simulink model "s8_10"  (Simulink 10.0)
settings: Solver=ode23  StartTime=0.0  StopTime=t_d  MaxStep=Tc  RelTol=1e-8  AbsTol=1e-8
values from neighbouring files (symbols this model uses):
  a = [1;1]    [MOTIONCONTROL.m]    (also in Robot_Maker.m = evalin('base', 'a'))
  F_v = K_r*diag([0.01 0.01])*K_r    [MOTIONCONTROL.m]
  g = [atan2d(r32,-r31);atan2d(sqrt(power(r13,2)+power(r23,2)),r33);atan2d(r23,r13)]    [DEMOGUI.m]    (also in MOTIONCONTROL.m = 9.81; invJacob_3axis.m = true; inverse_kinematics_Jac.m = true)
  K_d = 750*diag([1 1])    [MOTIONCONTROL.m]
  K_p = 375*diag([1 1])    [MOTIONCONTROL.m]
  pi_l = pi_m    [MOTIONCONTROL.m]
  q_d = [q1des q2des]    [MOTIONCONTROL.m]
  q_i = [q1ini q2ini]    [MOTIONCONTROL.m]
  Tc = 0.01    [MOTIONCONTROL.m]
  Ts = Tc    (= 0.01)    [MOTIONCONTROL.m]
undefined symbols (not defined in the file or in its folder): iner_l, pi_m
settings Model: Creator=luigivillani  LastModifiedBy=vivek  ExtModeAutoUpdateStatusClock=off
settings SolverCC: AutoScaleAbsTol=off  InitialStep=0.1*Tc
settings DataIOCC: SignalLoggingSaveFormat=ModelDataLogs  SaveOutput=off  SaveTime=off
settings OptimizationCC: BlockReduction=off  BooleanDataType=off  ExpressionDepthLimit=2147483647  InitFltsAndDblsToZero=on
settings DebuggingCC: SaveWithParameterizedLinksMsg=none  SignalResolutionControl=TryResolveAllWithWarning  MultiTaskDSMMsg=warning  MultiTaskCondExecSysMsg=none  FcnCallInpInsideContextMsg=warning  StateNameClashWarn=warning
settings HardwareCC: TargetUnknown=on
settings SFSimCC: SimUseLocalCustomCode=on  CustomCodeUndefinedFunction=FilterOut
settings RTWCC: RTWUseLocalCustomCode=on
settings GRTTargetCC: TargetFcnLib=ansi_tfl_tmw.mat

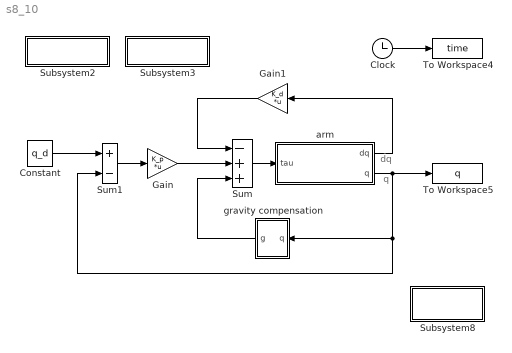
== system s8_10 ==
  note: dq
  note: q
  Clock : Clock
  Constant : Constant  Value=q_d
  Gain : Gain  Gain=K_p  Multiplication=Matrix(K*u)  SampleTime=Tc
      mask Display: disp('K_p')
  Gain1 : Gain  Gain=K_d  Multiplication=Matrix(K*u)  SampleTime=Tc
      mask Display: disp('K_d')
  Subsystem2 : Subsystem
      settings: OpenFcn=clear all;c=0;i8_10;
      mask Display: disp('q_d=[pi/4 -pi/2]')
  Subsystem3 : Subsystem
      settings: OpenFcn=clear all;c=1;i8_10;
      mask Display: disp('q_d=[-pi -3pi/4]')
  Subsystem8 : Subsystem
      settings: OpenFcn=p8_10;
      mask Display: disp('plot')
  Sum : Sum  Inputs=-++  SaturateOnIntegerOverflow=on  InputSameDT=on  OutDataTypeStr=Inherit: Same as first input
  Sum1 : Sum  Inputs=+-  SampleTime=Tc  SaturateOnIntegerOverflow=on  InputSameDT=on  OutDataTypeStr=Inherit: Same as first input
  To Workspace4 : ToWorkspace  VariableName=time  SampleTime=Ts
      settings: MaxDataPoints=4001
  To Workspace5 : ToWorkspace  VariableName=q  SampleTime=Ts
      settings: MaxDataPoints=4001
  arm : Subsystem
      mask Display: disp('inv(B(q))(tau-tau'')')
  gravity compensation : Subsystem
      mask Display: disp('g(q)')
  wires:
  Sum/1 -> arm/1(tau)
  arm/1(dq) -> Gain1/1
  Gain1/1 -> Sum/1
  Sum1/1 -> Gain/1
  Clock/1 -> To Workspace4/1
  Gain/1 -> Sum/2
  gravity compensation/1(g) -> Sum/3
  Constant/1 -> Sum1/1
  arm/2("q ") -> To Workspace5/1, Sum1/2, gravity compensation/1(q)

== system s8_10/Subsystem2 ==
  note: start

== system s8_10/Subsystem3 ==
  note: start

== system s8_10/Subsystem8 ==
  note: start

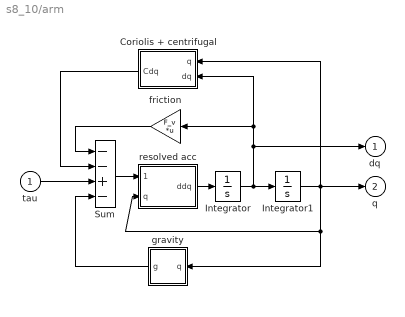
== system s8_10/arm ==
  tau : Inport
  Coriolis + centrifugal : Subsystem
      mask Display: disp('C(q,dq)dq')
  Integrator : Integrator  InitialCondition=[0 0]  ZeroCross=off
  Integrator1 : Integrator  InitialCondition=q_i  ZeroCross=off
  Sum : Sum  Inputs=--+-  SaturateOnIntegerOverflow=on  InputSameDT=on  OutDataTypeStr=Inherit: Same as first input
  friction : Gain  Gain=F_v  Multiplication=Matrix(K*u)  SaturateOnIntegerOverflow=on  OutDataTypeStr=Inherit: Same as input  ParamDataTypeStr=Inherit: Same as input
      mask Display: disp('F_v')
  gravity : Subsystem
      mask Display: disp('g(q)')
  resolved acc : Subsystem
      mask Display: disp('inv(B(q))')
  dq : Outport  InitialOutput=0
  "q " : Outport  Port=2  InitialOutput=0
  wires:
  Coriolis + centrifugal/1(Cdq) -> Sum/2
  tau/1 -> Sum/3
  Integrator1/1 -> Coriolis + centrifugal/1(q), resolved acc/2(q), gravity/1(q), "q "/1
  resolved acc/1(ddq) -> Integrator/1
  Integrator/1 -> Integrator1/1, dq/1, Coriolis + centrifugal/2(dq), friction/1
  Sum/1 -> resolved acc/1(tau-tau')
  friction/1 -> Sum/1
  gravity/1(g) -> Sum/4

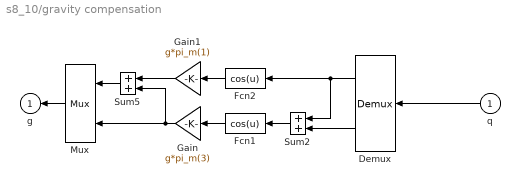
== system s8_10/gravity compensation ==
  q : Inport
  Demux : Demux  Outputs=2
  Fcn1 : Fcn  Expr=cos(u)  SampleTime=Tc
  Fcn2 : Fcn  Expr=cos(u)  SampleTime=Tc
  Gain : Gain  Gain=g*pi_m(3)  SaturateOnIntegerOverflow=on  OutDataTypeStr=Inherit: Same as input  ParamDataTypeStr=Inherit: Same as input
      mask Display: disp('k_2')
  Gain1 : Gain  Gain=g*pi_m(1)  SaturateOnIntegerOverflow=on  OutDataTypeStr=Inherit: Same as input  ParamDataTypeStr=Inherit: Same as input
      mask Display: disp('k_1')
  Mux : Mux  Inputs=2
  Sum2 : Sum  SampleTime=Tc  SaturateOnIntegerOverflow=on  InputSameDT=on  OutDataTypeStr=Inherit: Same as first input
  Sum5 : Sum  SaturateOnIntegerOverflow=on  InputSameDT=on  OutDataTypeStr=Inherit: Same as first input
  g : Outport  InitialOutput=0
  wires:
  Mux/1 -> g/1
  Gain/1 -> Sum5/2, Mux/2
  Sum5/1 -> Mux/1
  Gain1/1 -> Sum5/1
  Demux/1 -> Fcn2/1, Sum2/1
  Fcn2/1 -> Gain1/1
  Fcn1/1 -> Gain/1
  Sum2/1 -> Fcn1/1
  Demux/2 -> Sum2/2
  q/1 -> Demux/1

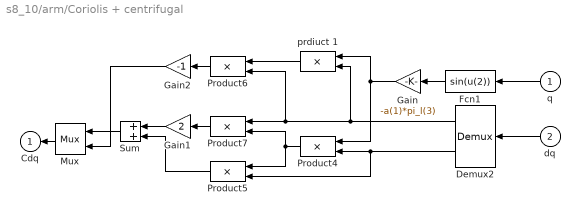
== system s8_10/arm/Coriolis + centrifugal ==
  q : Inport
  dq : Inport  Port=2
  Demux2 : Demux  Outputs=2
  Fcn1 : Fcn  Expr=sin(u(2))
  Gain : Gain  Gain=-a(1)*pi_l(3)  SaturateOnIntegerOverflow=on  OutDataTypeStr=Inherit: Same as input  ParamDataTypeStr=Inherit: Same as input
      mask Display: disp('k_3')
  Gain1 : Gain  Gain=2  SaturateOnIntegerOverflow=on  OutDataTypeStr=Inherit: Same as input  ParamDataTypeStr=Inherit: Same as input
  Gain2 : Gain  Gain=-1  SaturateOnIntegerOverflow=on  OutDataTypeStr=Inherit: Same as input  ParamDataTypeStr=Inherit: Same as input
  Mux : Mux  Inputs=2
  Product{4..7} (4 alike) : Product  SaturateOnIntegerOverflow=on  RndMeth=Zero  InputSameDT=on  OutDataTypeStr=Inherit: Same as first input
  Sum : Sum  SaturateOnIntegerOverflow=on  InputSameDT=on  OutDataTypeStr=Inherit: Same as first input
  prdiuct 1 : Product  SaturateOnIntegerOverflow=on  RndMeth=Zero  InputSameDT=on  OutDataTypeStr=Inherit: Same as first input
  Cdq : Outport  InitialOutput=0
  wires:
  dq/1 -> Demux2/1
  Gain2/1 -> Mux/2
  Product6/1 -> Gain2/1
  Mux/1 -> Cdq/1
  Sum/1 -> Mux/1
  Product5/1 -> Sum/2
  Gain1/1 -> Sum/1
  Product7/1 -> Gain1/1
  Demux2/1 -> prdiuct 1/2, Product6/2, Product7/1
  Demux2/2 -> Product4/2, Product5/2
  prdiuct 1/1 -> Product6/1
  Gain/1 -> prdiuct 1/1, Product4/1
  Fcn1/1 -> Gain/1
  q/1 -> Fcn1/1
  Product4/1 -> Product5/1, Product7/2

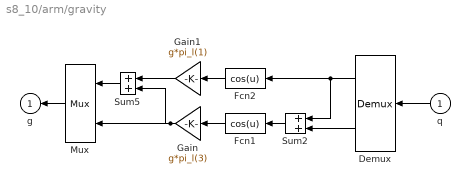
== system s8_10/arm/gravity ==
  q : Inport
  Demux : Demux  Outputs=2
  Fcn1 : Fcn  Expr=cos(u)
  Fcn2 : Fcn  Expr=cos(u)
  Gain : Gain  Gain=g*pi_l(3)  SaturateOnIntegerOverflow=on  OutDataTypeStr=Inherit: Same as input  ParamDataTypeStr=Inherit: Same as input
      mask Display: disp('k_2')
  Gain1 : Gain  Gain=g*pi_l(1)  SaturateOnIntegerOverflow=on  OutDataTypeStr=Inherit: Same as input  ParamDataTypeStr=Inherit: Same as input
      mask Display: disp('k_1')
  Mux : Mux  Inputs=2
  Sum2 : Sum  SaturateOnIntegerOverflow=on  InputSameDT=on  OutDataTypeStr=Inherit: Same as first input
  Sum5 : Sum  SaturateOnIntegerOverflow=on  InputSameDT=on  OutDataTypeStr=Inherit: Same as first input
  g : Outport  InitialOutput=0
  wires:
  q/1 -> Demux/1
  Demux/2 -> Sum2/2
  Sum2/1 -> Fcn1/1
  Fcn1/1 -> Gain/1
  Fcn2/1 -> Gain1/1
  Demux/1 -> Fcn2/1, Sum2/1
  Gain1/1 -> Sum5/1
  Sum5/1 -> Mux/1
  Gain/1 -> Sum5/2, Mux/2
  Mux/1 -> g/1

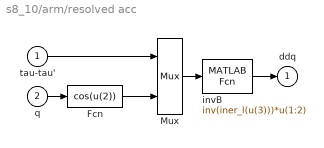
== system s8_10/arm/resolved acc ==
  tau-tau' : Inport
  q : Inport  Port=2
  Fcn : Fcn  Expr=cos(u(2))
  Mux : Mux  Inputs=[2,1]
  "invB " : MATLABFcn  MATLABFcn=inv(iner_l(u(3)))*u(1:2)  OutputDimensions=2
      mask Display: disp('inv(B(q))')
  ddq : Outport  InitialOutput=0
  wires:
  Fcn/1 -> Mux/2
  q/1 -> Fcn/1
  "invB "/1 -> ddq/1
  tau-tau'/1 -> Mux/1
  Mux/1 -> "invB "/1
